simulink model "vocoder"  (R2020a)
settings: Solver=FixedStepDiscrete  StartTime=0.0  StopTime=inf  RelTol=1e-3
libraries: dspvision x3, dspstat3 x1
settings Model: Creator=unity  LastModifiedBy=unity
settings SolverCC: AutoInsertRateTranBlk=on
settings DataIOCC: LimitDataPoints=on  SaveOutput=off  SignalLogging=off  SaveTime=off
settings OptimizationCC: LifeSpan=inf
settings DebuggingCC: AlgebraicLoopMsg=error  SingleTaskRateTransMsg=error  AllowSymbolicDim=off  SFUnexpectedBacktrackingDiag=warning  SFNoUnconditionalDefaultTransitionDiag=warning  SFExecutionAtInitializationDiag=none  UnderSpecifiedDimensionMsg=warning  ArithmeticOperatorsInVariantConditions=warning
settings SFSimCC: SimUseLocalCustomCode=off  CustomCodeUndefinedFunction=UseInterfaceOnly
settings RTWCC: RTWUseLocalCustomCode=off
settings CodeAppCC: StateflowObjectComments=on
settings GRTTargetCC: TargetLangStandard=C89/C90 (ANSI)
settings ConfigComp: CovMetricSettings=dw  CovHtmlReporting=on  CovSaveCumulativeToWorkspaceVar=on  CovSaveSingleToWorkspaceVar=on  CovExternalEMLEnable=off  CovSFcnEnable=off

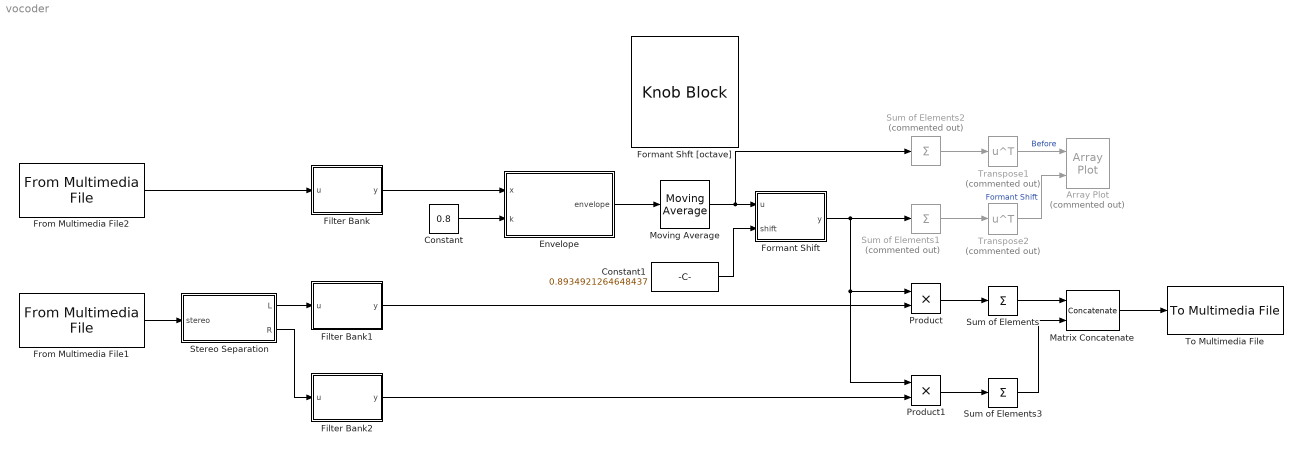
== system vocoder ==
  Array Plot : ArrayPlot  Commented=on  NumInputPorts=2
  Constant : Constant  Value=0.8
  Constant1 : Constant  Value=0.8934921264648437
  Envelope : MATLAB Function  TreatAsAtomicUnit=on
  Filter Bank : MATLAB Function  TreatAsAtomicUnit=on
  Filter Bank1 : MATLAB Function  TreatAsAtomicUnit=on
  Filter Bank2 : MATLAB Function  TreatAsAtomicUnit=on
  Formant Shft [octave] : KnobBlock  ScaleMin=-3  ScaleMax=3
  Formant Shift : MATLAB Function  TreatAsAtomicUnit=on
  From Multimedia File1 : dspvision/From Multimedia File  inputFilename=D:\github\matlab_audio\qiita\03_vocoder\audio_resource\stereo_synth.wav  readRange=[1 Inf]  loop=on  numPlays=1  outputStreams=オーディオのみ  videoDataType=single  audioDataType=double  inheritSampleTime=on  userDefinedSampleTime=1/30  noAudioOutput=off  isIntensityVideo=off  fourcc=RGB  colorVideoFormat=Separate color signals  outputEOF=off  dataOrg=Column-major  audioFrameSize=1024  computeAudioFrameSize=off  outSamplingMode=Sample based
  From Multimedia File2 : dspvision/From Multimedia File  inputFilename=D:\github\matlab_audio\qiita\03_vocoder\audio_resource\stereo.wav  readRange=[1 Inf]  loop=on  numPlays=1  outputStreams=オーディオのみ  videoDataType=single  audioDataType=double  inheritSampleTime=on  userDefinedSampleTime=1/30  noAudioOutput=off  isIntensityVideo=off  fourcc=RGB  colorVideoFormat=Separate color signals  outputEOF=off  dataOrg=Column-major  audioFrameSize=1024  computeAudioFrameSize=off  outSamplingMode=Sample based
  Matrix Concatenate : Concatenate  Mode=Multidimensional array  ConcatenateDimension=2
  Moving Average : dspstat3/Moving Average  Method=Sliding window  ForgettingFactorPort=off  SpecifyWindowLength=on  WindowLength=500  ForgettingFactor=0.9  SimulateUsing=Code generation
  Product : Product
  Product1 : Product
  Stereo Separation : MATLAB Function  TreatAsAtomicUnit=on
  Sum of Elements : Sum  Inputs=+  CollapseMode=Specified dimension  CollapseDim=2
  Sum of Elements1 : Sum  Commented=on  Inputs=+  CollapseMode=Specified dimension
  Sum of Elements2 : Sum  Commented=on  Inputs=+  CollapseMode=Specified dimension
  Sum of Elements3 : Sum  Inputs=+  CollapseMode=Specified dimension  CollapseDim=2
  To Multimedia File : dspvision/To Multimedia File  outputFilename=output.wav  streamSelection=Audio only  videoCompressor=None (uncompressed)  audioCompressor=None (uncompressed)  imagePorts=Separate color signals  fileType=WAV  audioDatatype=16-bit integer  fourcc=RGB  videoQuality=75  mj2000CompFactor=10
  Transpose1 : Math  Commented=on  Operator=transpose  SaturateOnIntegerOverflow=on
  Transpose2 : Math  Commented=on  Operator=transpose  SaturateOnIntegerOverflow=on
  wires:
  From Multimedia File2/1 -> Filter Bank/1(u)
  Filter Bank/1(y) -> Envelope/1(x)
  Constant/1 -> Envelope/2(k)
  Envelope/1(envelope) -> Moving Average/1
  Filter Bank1/1(y) -> Product/2
  Moving Average/1 -> Sum of Elements2/1, Formant Shift/1(u)
  Product/1 -> Sum of Elements/1
  Sum of Elements1/1 -> Transpose2/1
  Transpose2/1 -> Array Plot/2  "Formant Shift"
  Formant Shift/1(y) -> Sum of Elements1/1, Product1/1, Product/1
  Transpose1/1 -> Array Plot/1  "Before"
  Sum of Elements2/1 -> Transpose1/1
  Constant1/1 -> Formant Shift/2(shift)
  Filter Bank2/1(y) -> Product1/2
  Stereo Separation/2(R) -> Filter Bank2/1(u)
  Sum of Elements/1 -> Matrix Concatenate/1
  Sum of Elements3/1 -> Matrix Concatenate/2
  Matrix Concatenate/1 -> To Multimedia File/1
  Product1/1 -> Sum of Elements3/1
  From Multimedia File1/1 -> Stereo Separation/1(stereo)
  Stereo Separation/1(L) -> Filter Bank1/1(u)

== matlab function vocoder/Filter Bank ==
  data: u input; y output
function y = fcn(u)
    %フィルタバンクオブジェクトの作成
    persistent ofb
    if isempty(ofb)
        ofb = octaveFilterBank('1/48 octave',"FilterOrder",2);
    end

    %フィルタバンクの適用
    y = ofb(u);

== matlab function vocoder/Filter Bank1 ==
  data: u input; y output
function y = fcn(u)
    %フィルタバンクオブジェクトの作成
    persistent ofb
    if isempty(ofb)
        ofb = octaveFilterBank('1/48 octave',"FilterOrder",2);
    end

    %フィルタバンクの適用
    y = ofb(u);

== matlab function vocoder/Formant Shift ==
  data: u input; y output; shift input
function y  = fcn(u,shift)
    %フレームサイズと帯域の分割数を取得
    [frame_size,n_bands]=size(u);
    
    %エンヴェロープの左右に余白を取る（エンヴェロープの配列と同じ大きさのゼロ行列を結合）
    v = cat(2,cat(2,zeros(frame_size,n_bands),u),zeros(frame_size,n_bands));
    
    %フォルマントシフト後の配列の始めの要素が，フォルマントシフト前のどの要素だったのかを取得
    %余白を取った分，n_bandsだけ平行移動している
    %オクターブフィルタが1/6 octaveなので，6を掛けて単位をオクターブにそろえる
    %マトラボでは始めの要素は１なので，１を足す
    p = n_bands-shift*6+1;
    
    %整数部分の計算
    p_int = floor(p);
    
    %小数部分の計算
    p_dec = p - p_int;
    
    %二つの配列のブレンド
    y = v(:,(p_int):(p_int+n_bands-1))*(1-p_dec)+v(:,(p_int+1):(p_int+n_bands))*p_dec;

== matlab function vocoder/Filter Bank2 ==
  data: u input; y output
function y = fcn(u)
    %フィルタバンクオブジェクトの作成
    persistent ofb
    if isempty(ofb)
        ofb = octaveFilterBank('1/48 octave',"FilterOrder",2);
    end

    %フィルタバンクの適用
    y = ofb(u);

== matlab function vocoder/Stereo Separation ==
  data: stereo input; L output; R output
function [L,R] = fcn(stereo)
    L = stereo(:,1);
    R = stereo(:,2);

== matlab function vocoder/Envelope ==
  data: x input; envelope output; k input
function envelope = fcn(x,k)
    %入力の配列のサイズから帯域数n_bandsとframe_sizeを求める
    [n_bands,frame_size]=size(x);

    %現在のエンヴェロープの値を保存する永続な配列yの作成
    persistent y
    if isempty(y)
        y = zeros(n_bands);
    end

    %入力の絶対値を取る
    x = abs(x);

    %エンヴェロープの配列の初期化
    envelope = zeros(n_bands,frame_size);

    %全体域にわたる繰り返し
    for band = 1:n_bands
        %全サンプルにわたる繰り返し
        for i = 1:frame_size
            %yの値の更新
            if y(band) <= x(band,i)
                y(band) = x(band,i);
            else
                y(band) = y(band)*k;
            end
            envelope(band,i) = y(band);
        end
    end
end
